simulink model "Events2"  (Simulink 8.7)
settings: Solver=ode45  StartTime=0.0  StopTime=10.0  RelTol=1e-3
settings Model: Creator=scaife  LastModifiedBy=hamza  ExtModeAutoUpdateStatusClock=off
settings DataIOCC: SignalLoggingSaveFormat=ModelDataLogs  SignalLoggingName=sigsOut
settings DebuggingCC: SaveWithParameterizedLinksMsg=none  SignalResolutionControl=TryResolveAllWithWarning  MultiTaskDSMMsg=warning  MultiTaskCondExecSysMsg=none  StrictBusMsg=None
settings HardwareCC: TargetUnknown=on
settings SFSimCC: SimParseCustomCode=off
settings GRTTargetCC: GeneratePreprocessorConditionals=Use local settings  CombineOutputUpdateFcns=off  GRTInterface=on

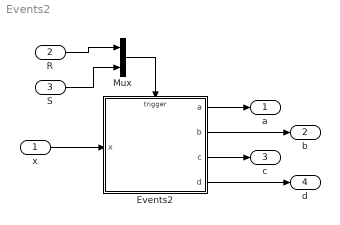
== system Events2 ==
  x : Inport
  R : Inport  Port=2
  S : Inport  Port=3
  Events2 : Stateflow chart  TreatAsAtomicUnit=on
  Mux : Mux  Inputs=2
  a : Outport
  b : Outport  Port=2
  c : Outport  Port=3
  d : Outport  Port=4
  wires:
  x/1 -> Events2/1(x)
  Mux/1 -> Events2/Trigger
  R/1 -> Mux/1
  S/1 -> Mux/2
  Events2/1(a) -> a/1
  Events2/2(b) -> b/1
  Events2/3(c) -> c/1
  Events2/4(d) -> d/1

== stateflow chart Events2 ==
  state B [parallel]
    settings: executionOrder=2
    state Ba/
      en:b=x+3
    state Bb/
      en:b=x+4
    (default) -> Ba
    Ba -> Bb : S1/send(S2,C)
    Bb -> Ba : R1/send(R2,C)
  state A [parallel]
    settings: executionOrder=1
    state Aa/
      en:a=x+1
    state Ab/
      en:a=x+2
    (default) -> Aa
    Aa -> Ab : S/send(S1,B)
    Ab -> Aa : R/send(R1,B)
  state D [parallel]
    settings: executionOrder=4
    state Da/
      en:d=x+7
    state Db/
      en:d=x+8
    (default) -> Da
    Da -> Db : S3
    Db -> Da : R3
  state C [parallel]
    settings: executionOrder=3
    state Cb/
      en:c=x+6
    state Ca/
      en:c=x+5
    (default) -> Ca
    Ca -> Cb : S2/send(S3,D)
    Cb -> Ca : R2/send(R3,D)
  data: a output int32; x input int32; b output int32; c output int32; d output int32
  events: R1 local EITHER_EDGE_EVENT; S1 local EITHER_EDGE_EVENT; R input EITHER_EDGE_EVENT; S input EITHER_EDGE_EVENT; R2 local EITHER_EDGE_EVENT; S2 local EITHER_EDGE_EVENT; S3 local EITHER_EDGE_EVENT; R3 local EITHER_EDGE_EVENT
